simulink model "open_mha"  (R2020b)
settings: Solver=FixedStepAuto  StartTime=0.0  StopTime=stopTime  RelTol=1e-3
InitFcn:
  | initCallback
StopFcn:
  | stopCallback
values from neighbouring files (symbols this model uses):
  attack_decay_data_default_value = 1048576    [modelparameters.m]
  gain_table_default_data = 16711680    [modelparameters.m]
undefined symbols (not defined in the file or in its folder): mp
settings Model: DataTypeOverride=Off  SimulationMode=accelerator  Creator=Ross  LastModifiedBy=conno
settings SolverCC: AutoInsertRateTranBlk=on
settings DataIOCC: ReturnWorkspaceOutputs=off
settings OptimizationCC: BlockReduction=off  ConditionallyExecuteInputs=off  DefaultParameterBehavior=Inlined
settings DebuggingCC: ReadBeforeWriteMsg=DisableAll  WriteAfterWriteMsg=DisableAll  WriteAfterReadMsg=DisableAll  AlgebraicLoopMsg=error  MultiTaskDSMMsg=none  SingleTaskRateTransMsg=error  PregeneratedLibrarySubsystemCodeDiagnostic=none  ArithmeticOperatorsInVariantConditions=warning
settings HardwareCC: ProdBitPerPointer=32  ProdBitPerSizeT=32  ProdBitPerPtrDiffT=32  ProdLargestAtomicFloat=None  ProdIntDivRoundTo=Undefined  ProdEndianess=Unspecified  ProdWordSize=32  ProdHWDeviceType=ASIC/FPGA->ASIC/FPGA  TargetBitPerPointer=64  TargetBitPerSizeT=64  TargetBitPerPtrDiffT=64  TargetLongLongMode=on  TargetIntDivRoundTo=Zero  TargetEndianess=LittleEndian  TargetWordSize=64  TargetHWDeviceType=Custom Processor->MATLAB Host Computer  ProdEqTarget=off
settings ModelReferenceCC: UpdateModelReferenceTargets=IfOutOfDate  EnableParallelModelReferenceBuilds=on  ParallelModelReferenceMATLABWorkerInit=Copy Base Workspace
settings SFSimCC: SFSimEcho=off  SimUseLocalCustomCode=off  CustomCodeUndefinedFunction=UseInterfaceOnly
settings RTWCC: RTWUseLocalCustomCode=off

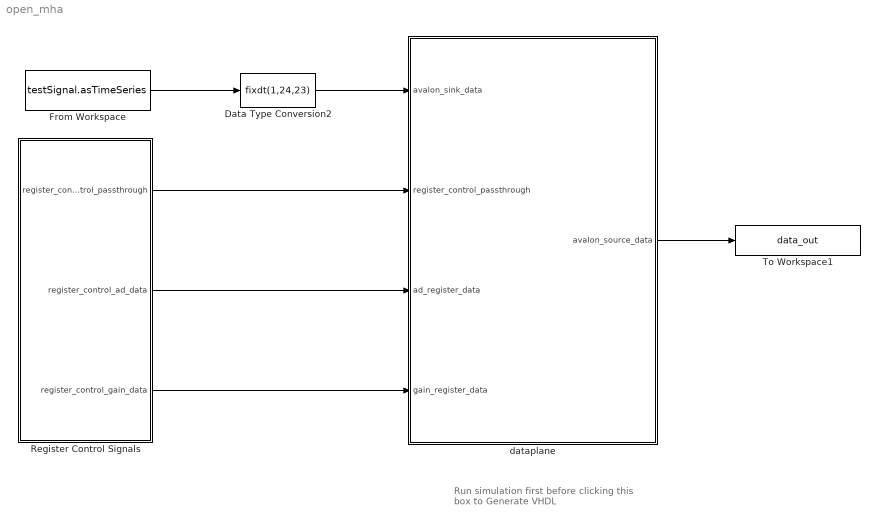
== system open_mha ==
  note: Run simulation first
      | before clicking this box to
      | Generate VHDL
  Data Type Conversion2 : DataTypeConversion  OutDataTypeStr=fixdt(1,24,23)
  From Workspace : FromWorkspace  VariableName=testSignal.asTimeSeries  SampleTime=mp.Ts
  Register Control Signals : Subsystem
  To Workspace1 : ToWorkspace  VariableName=data_out  SampleTime=-1
  dataplane : Subsystem  TreatAsAtomicUnit=on
  wires:
  dataplane/1("avalon_source_data ") -> To Workspace1/1
  Register Control Signals/1(register_control_passthrough) -> dataplane/2(register_control_passthrough)
  From Workspace/1 -> Data Type Conversion2/1
  Data Type Conversion2/1 -> dataplane/1(avalon_sink_data)
  Register Control Signals/2("register_control_ad_data ") -> dataplane/3(ad_register_data)
  Register Control Signals/3(register_control_gain_data) -> dataplane/4(gain_register_data)

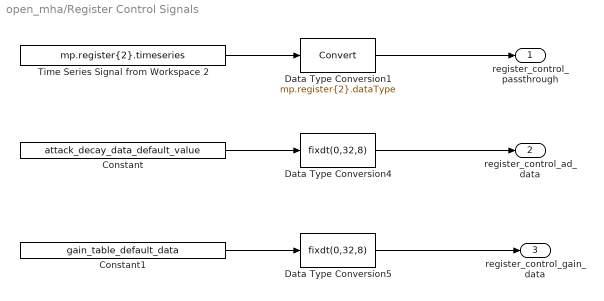
== system open_mha/Register Control Signals ==
  Constant : Constant  Value=attack_decay_data_default_value  SampleTime=mp.Ts
  Constant1 : Constant  Value=gain_table_default_data  SampleTime=mp.Ts
  Data Type Conversion1 : DataTypeConversion  OutDataTypeStr=mp.register{2}.dataType  RndMeth=Nearest
  Data Type Conversion4 : DataTypeConversion  OutDataTypeStr=fixdt(0,32,8)
  Data Type Conversion5 : DataTypeConversion  OutDataTypeStr=fixdt(0,32,8)
  Time Series Signal from Workspace 2 : FromWorkspace  VariableName=mp.register{2}.timeseries  OutDataTypeStr=double  SampleTime=mp.Ts  OutputAfterFinalValue=Holding final value
  register_control_passthrough : Outport  VectorParamsAs1DForOutWhenUnconnected=off
  "register_control_ad_data " : Outport  Port=2  VectorParamsAs1DForOutWhenUnconnected=off
  register_control_gain_data : Outport  Port=3  VectorParamsAs1DForOutWhenUnconnected=off
  wires:
  Time Series Signal from Workspace 2/1 -> Data Type Conversion1/1
  Data Type Conversion1/1 -> register_control_passthrough/1
  Data Type Conversion5/1 -> register_control_gain_data/1
  Data Type Conversion4/1 -> "register_control_ad_data "/1
  Constant/1 -> Data Type Conversion4/1
  Constant1/1 -> Data Type Conversion5/1

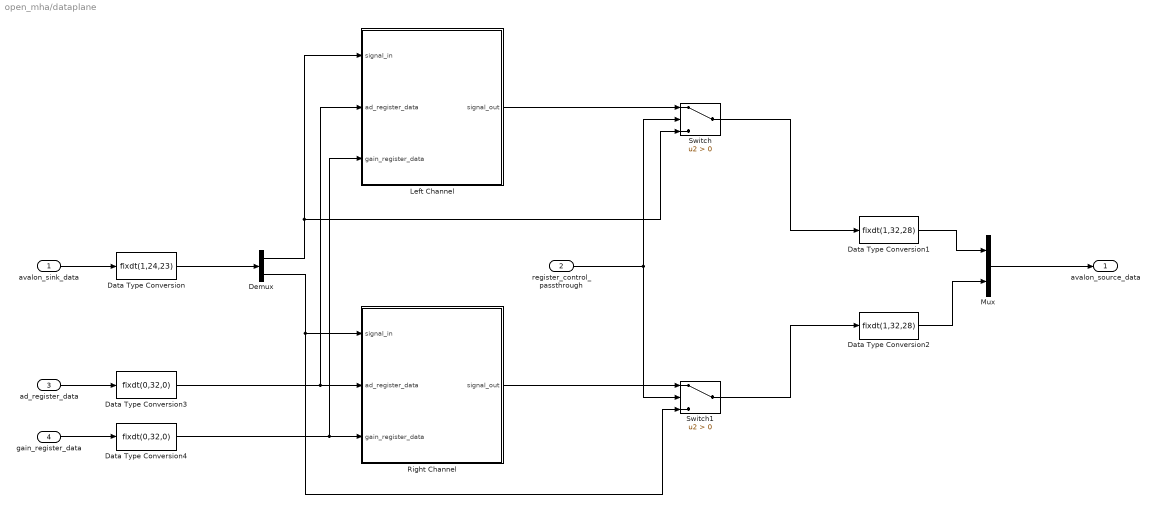
== system open_mha/dataplane ==
  avalon_sink_data : Inport
  register_control_passthrough : Inport  Port=2
  ad_register_data : Inport  Port=3
  gain_register_data : Inport  Port=4
  Data Type Conversion : DataTypeConversion  OutDataTypeStr=fixdt(1,24,23)
  Data Type Conversion1 : DataTypeConversion  OutDataTypeStr=fixdt(1,32,28)
  Data Type Conversion2 : DataTypeConversion  OutDataTypeStr=fixdt(1,32,28)
  Data Type Conversion3 : DataTypeConversion  OutDataTypeStr=fixdt(0,32,0)  ConvertRealWorld=Stored Integer (SI)
  Data Type Conversion4 : DataTypeConversion  OutDataTypeStr=fixdt(0,32,0)  ConvertRealWorld=Stored Integer (SI)
  Demux : Demux  Outputs=2
  Left Channel : Subsystem  TreatAsAtomicUnit=on
  Mux : Mux  Inputs=2
  Right Channel : Subsystem  TreatAsAtomicUnit=on
  Switch : Switch  Criteria=u2 > Threshold
  Switch1 : Switch  Criteria=u2 > Threshold
  "avalon_source_data " : Outport  InitialOutput=0  VectorParamsAs1DForOutWhenUnconnected=off
  wires:
  avalon_sink_data/1 -> Data Type Conversion/1
  Demux/1 -> Left Channel/1(signal_in), Switch/3
  Data Type Conversion1/1 -> Mux/1
  Data Type Conversion2/1 -> Mux/2
  Mux/1 -> "avalon_source_data "/1
  register_control_passthrough/1 -> Switch/2, Switch1/2
  Data Type Conversion/1 -> Demux/1
  Demux/2 -> Right Channel/1(signal_in), Switch1/3
  Switch/1 -> Data Type Conversion1/1
  Switch1/1 -> Data Type Conversion2/1
  ad_register_data/1 -> Data Type Conversion3/1
  gain_register_data/1 -> Data Type Conversion4/1
  Left Channel/1(signal_out) -> Switch/1
  Right Channel/1(signal_out) -> Switch1/1
  Data Type Conversion3/1 -> Right Channel/2(ad_register_data), Left Channel/2(ad_register_data)
  Data Type Conversion4/1 -> Right Channel/3(gain_register_data), Left Channel/3(gain_register_data)

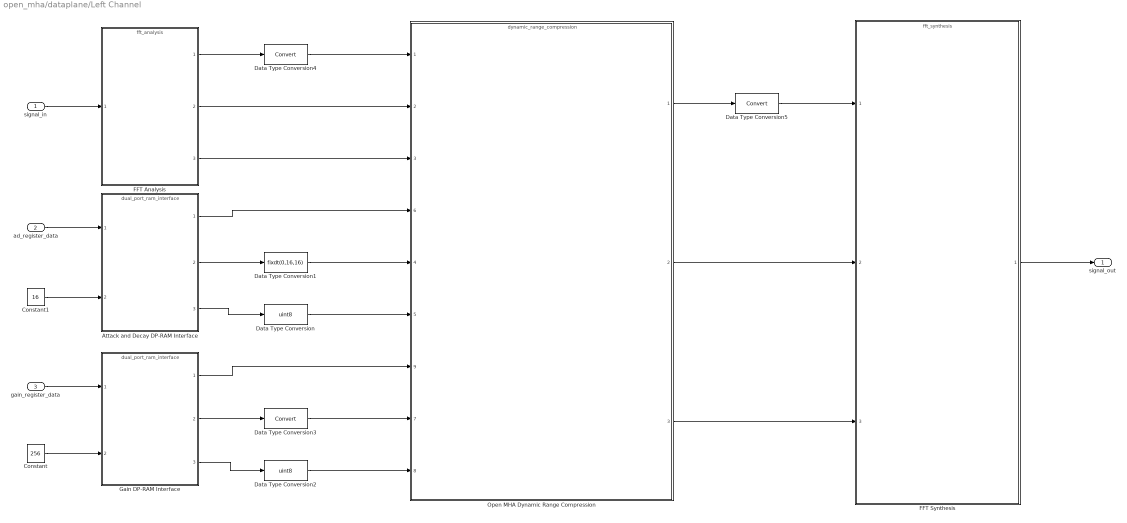
== system open_mha/dataplane/Left Channel ==
  signal_in : Inport
  ad_register_data : Inport  Port=2
  gain_register_data : Inport  Port=3
  Attack and Decay DP-RAM Interface : ModelReference  ModelNameDialog=dual_port_ram_interface.slx  SimulationMode=Normal  ModelReferenceVersion=1.113
  Constant : Constant  Value=256  OutDataTypeStr=Inherit: Inherit via back propagation  SampleTime=-1
  Constant1 : Constant  Value=16  OutDataTypeStr=Inherit: Inherit via back propagation  SampleTime=-1
  Data Type Conversion : DataTypeConversion  OutDataTypeStr=uint8
  Data Type Conversion1 : DataTypeConversion  OutDataTypeStr=fixdt(0,16,16)  ConvertRealWorld=Stored Integer (SI)
  Data Type Conversion2 : DataTypeConversion  OutDataTypeStr=uint8
  Data Type Conversion3 : DataTypeConversion  ConvertRealWorld=Stored Integer (SI)
  Data Type Conversion4 : DataTypeConversion
  Data Type Conversion5 : DataTypeConversion
  FFT Analysis : ModelReference  ModelNameDialog=fft_analysis.slx  SimulationMode=Normal  ModelReferenceVersion=1.150
  FFT Synthesis : ModelReference  ModelNameDialog=fft_synthesis.slx  SimulationMode=Normal  ModelReferenceVersion=3.6
  Gain DP-RAM Interface : ModelReference  ModelNameDialog=dual_port_ram_interface  SimulationMode=Normal  ModelReferenceVersion=1.113
  Open MHA Dynamic Range Compression : ModelReference  ModelNameDialog=dynamic_range_compression.slx  SimulationMode=Normal  ModelReferenceVersion=2.61
      settings: PortSchema="{\"entries\":[{\"content\":{\"sides\":[{\"content\":{\"connectorIds\":[\"In1\",\"In2\",\"In3\",\"In6\",\"In4\",\"In5\",\"In9\",\"In7\",\"In8\"]},\"type\":\"ConnectorPlacement.EquallySpacedRectSide\",\"uuid\":\"7bd236ff-1e1e-4fa4-89d0-719ac5007e48\"},{\"content\":{\"connectorIds\":[\"Out1\",\"Out2\",\"Out3\"],\"side\":\"RIGHT\"},\"type\":\"ConnectorPlacement.EquallySpacedRectSide\",\"uuid\":\"7bab585e-5b2f-4616-9cd3-d0f4391371e3\"},{\"content\":{\"connectorIds\":[],\"side\":\"TOP\"},\"type\":\"ConnectorPlacement.EquallySpacedRectSide\",\"uuid\":\"c11f42ca-01d0-46f7-9e57-80284b7f5bfd\"},{\"content\":{\"connectorIds\":[],\"side\":\"HIDDEN\"},\"type\":\"ConnectorPlacement.EquallySpacedRectSide\",\"uuid\":\"2205d400-6367-4424-a308-b45796d09249\"}]},\"type\":\"ConnectorPlacement.EquallySpacedConnector\",\"uuid\":\"c897d5ce-98de-4a61-878e-4201a99bc038\"}],\"packageUris\":[\"http://schema.mathworks.com/mf0/Connector/R2020b\"],\"version\":\"1.0\"}"
  signal_out : Outport  VectorParamsAs1DForOutWhenUnconnected=off
  wires:
  signal_in/1 -> FFT Analysis/1
  FFT Synthesis/1 -> signal_out/1
  FFT Analysis/1 -> Data Type Conversion4/1
  FFT Analysis/2 -> Open MHA Dynamic Range Compression/2
  Open MHA Dynamic Range Compression/2 -> FFT Synthesis/2
  Open MHA Dynamic Range Compression/3 -> FFT Synthesis/3
  Constant/1 -> Gain DP-RAM Interface/2
  gain_register_data/1 -> Gain DP-RAM Interface/1
  Constant1/1 -> Attack and Decay DP-RAM Interface/2
  ad_register_data/1 -> Attack and Decay DP-RAM Interface/1
  Attack and Decay DP-RAM Interface/2 -> Data Type Conversion1/1
  Attack and Decay DP-RAM Interface/3 -> Data Type Conversion/1
  Gain DP-RAM Interface/3 -> Data Type Conversion2/1
  Gain DP-RAM Interface/2 -> Data Type Conversion3/1
  Data Type Conversion4/1 -> Open MHA Dynamic Range Compression/1
  Data Type Conversion5/1 -> FFT Synthesis/1
  FFT Analysis/3 -> Open MHA Dynamic Range Compression/3
  Open MHA Dynamic Range Compression/1 -> Data Type Conversion5/1
  Attack and Decay DP-RAM Interface/1 -> Open MHA Dynamic Range Compression/6
  Gain DP-RAM Interface/1 -> Open MHA Dynamic Range Compression/9
  Data Type Conversion1/1 -> Open MHA Dynamic Range Compression/4
  Data Type Conversion/1 -> Open MHA Dynamic Range Compression/5
  Data Type Conversion3/1 -> Open MHA Dynamic Range Compression/7
  Data Type Conversion2/1 -> Open MHA Dynamic Range Compression/8

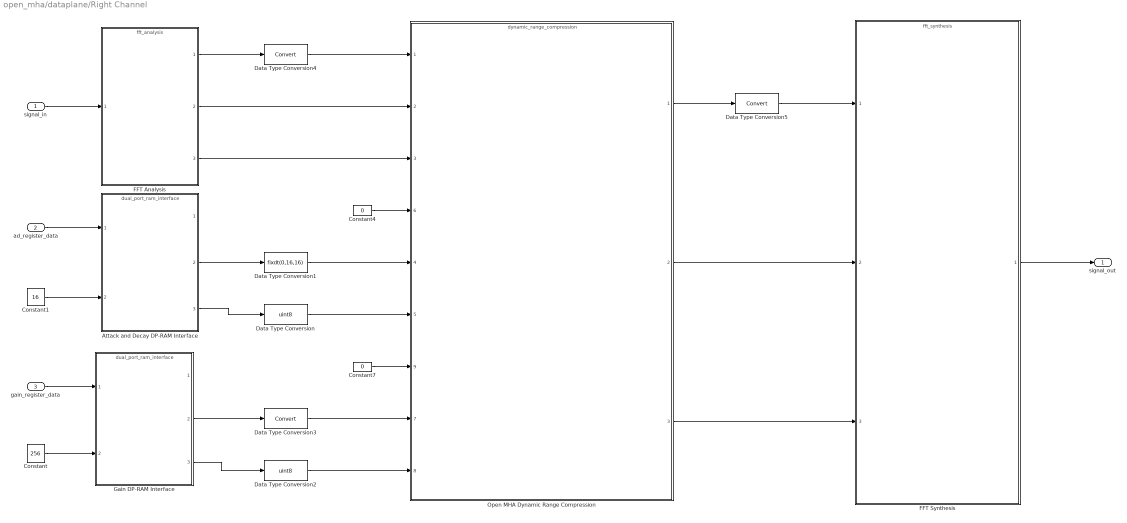
== system open_mha/dataplane/Right Channel ==
  signal_in : Inport
  ad_register_data : Inport  Port=2
  gain_register_data : Inport  Port=3
  Attack and Decay DP-RAM Interface : ModelReference  ModelNameDialog=dual_port_ram_interface  SimulationMode=Normal  ModelReferenceVersion=1.113
  Constant : Constant  Value=256  OutDataTypeStr=Inherit: Inherit via back propagation  SampleTime=-1
  Constant1 : Constant  Value=16  OutDataTypeStr=Inherit: Inherit via back propagation  SampleTime=-1
  Constant4 : Constant  Value=0  OutDataTypeStr=boolean  SampleTime=-1
  Constant7 : Constant  Value=0  OutDataTypeStr=boolean  SampleTime=-1
  Data Type Conversion : DataTypeConversion  OutDataTypeStr=uint8
  Data Type Conversion1 : DataTypeConversion  OutDataTypeStr=fixdt(0,16,16)  ConvertRealWorld=Stored Integer (SI)
  Data Type Conversion2 : DataTypeConversion  OutDataTypeStr=uint8
  Data Type Conversion3 : DataTypeConversion  ConvertRealWorld=Stored Integer (SI)
  Data Type Conversion4 : DataTypeConversion
  Data Type Conversion5 : DataTypeConversion
  FFT Analysis : ModelReference  ModelNameDialog=fft_analysis.slx  SimulationMode=Normal  ModelReferenceVersion=1.150
  FFT Synthesis : ModelReference  ModelNameDialog=fft_synthesis.slx  SimulationMode=Normal  ModelReferenceVersion=3.6
  Gain DP-RAM Interface : ModelReference  ModelNameDialog=dual_port_ram_interface  SimulationMode=Normal  ModelReferenceVersion=1.113
  Open MHA Dynamic Range Compression : ModelReference  ModelNameDialog=dynamic_range_compression.slx  SimulationMode=Normal  ModelReferenceVersion=2.61
      settings: PortSchema="{\"entries\":[{\"content\":{\"sides\":[{\"content\":{\"connectorIds\":[\"In1\",\"In2\",\"In3\",\"In6\",\"In4\",\"In5\",\"In9\",\"In7\",\"In8\"]},\"type\":\"ConnectorPlacement.EquallySpacedRectSide\",\"uuid\":\"7bd236ff-1e1e-4fa4-89d0-719ac5007e48\"},{\"content\":{\"connectorIds\":[\"Out1\",\"Out2\",\"Out3\"],\"side\":\"RIGHT\"},\"type\":\"ConnectorPlacement.EquallySpacedRectSide\",\"uuid\":\"7bab585e-5b2f-4616-9cd3-d0f4391371e3\"},{\"content\":{\"connectorIds\":[],\"side\":\"TOP\"},\"type\":\"ConnectorPlacement.EquallySpacedRectSide\",\"uuid\":\"c11f42ca-01d0-46f7-9e57-80284b7f5bfd\"},{\"content\":{\"connectorIds\":[],\"side\":\"HIDDEN\"},\"type\":\"ConnectorPlacement.EquallySpacedRectSide\",\"uuid\":\"2205d400-6367-4424-a308-b45796d09249\"}]},\"type\":\"ConnectorPlacement.EquallySpacedConnector\",\"uuid\":\"c897d5ce-98de-4a61-878e-4201a99bc038\"}],\"packageUris\":[\"http://schema.mathworks.com/mf0/Connector/R2020b\"],\"version\":\"1.0\"}"
  signal_out : Outport  VectorParamsAs1DForOutWhenUnconnected=off
  wires:
  signal_in/1 -> FFT Analysis/1
  FFT Synthesis/1 -> signal_out/1
  FFT Analysis/1 -> Data Type Conversion4/1
  FFT Analysis/2 -> Open MHA Dynamic Range Compression/2
  Open MHA Dynamic Range Compression/2 -> FFT Synthesis/2
  Open MHA Dynamic Range Compression/3 -> FFT Synthesis/3
  Constant/1 -> Gain DP-RAM Interface/2
  gain_register_data/1 -> Gain DP-RAM Interface/1
  Constant1/1 -> Attack and Decay DP-RAM Interface/2
  ad_register_data/1 -> Attack and Decay DP-RAM Interface/1
  Attack and Decay DP-RAM Interface/2 -> Data Type Conversion1/1
  Attack and Decay DP-RAM Interface/3 -> Data Type Conversion/1
  Gain DP-RAM Interface/3 -> Data Type Conversion2/1
  Gain DP-RAM Interface/2 -> Data Type Conversion3/1
  Data Type Conversion4/1 -> Open MHA Dynamic Range Compression/1
  Data Type Conversion5/1 -> FFT Synthesis/1
  FFT Analysis/3 -> Open MHA Dynamic Range Compression/3
  Open MHA Dynamic Range Compression/1 -> Data Type Conversion5/1
  Constant4/1 -> Open MHA Dynamic Range Compression/6
  Constant7/1 -> Open MHA Dynamic Range Compression/9
  Data Type Conversion1/1 -> Open MHA Dynamic Range Compression/4
  Data Type Conversion/1 -> Open MHA Dynamic Range Compression/5
  Data Type Conversion3/1 -> Open MHA Dynamic Range Compression/7
  Data Type Conversion2/1 -> Open MHA Dynamic Range Compression/8
